simulink model "test1my"  (R2024b)
settings: Solver=VariableStepAuto  StartTime=0.0  StopTime=0.5  RelTol=1e-3
undefined symbols (not defined in the file): Ion, Lithium
libraries: spsSeriesRLCBranchLib x7, spsVoltageMeasurementLib x5, spsMosfetLib x3, spsCurrentMeasurementLib x2, spsPVArrayLib x2, spsBatteryLib x1, spsBreakerLib x1, spsDiodeLib x1, slpidlib x1, spsTriangleGeneratorLib x1, sps_lib x1
settings Model: Creator=pansi  LastModifiedBy=ASUS

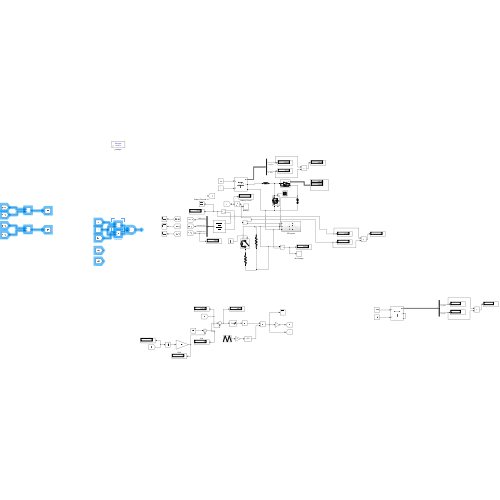
[thumbnail: Simulink's stored preview of the top-level diagram]
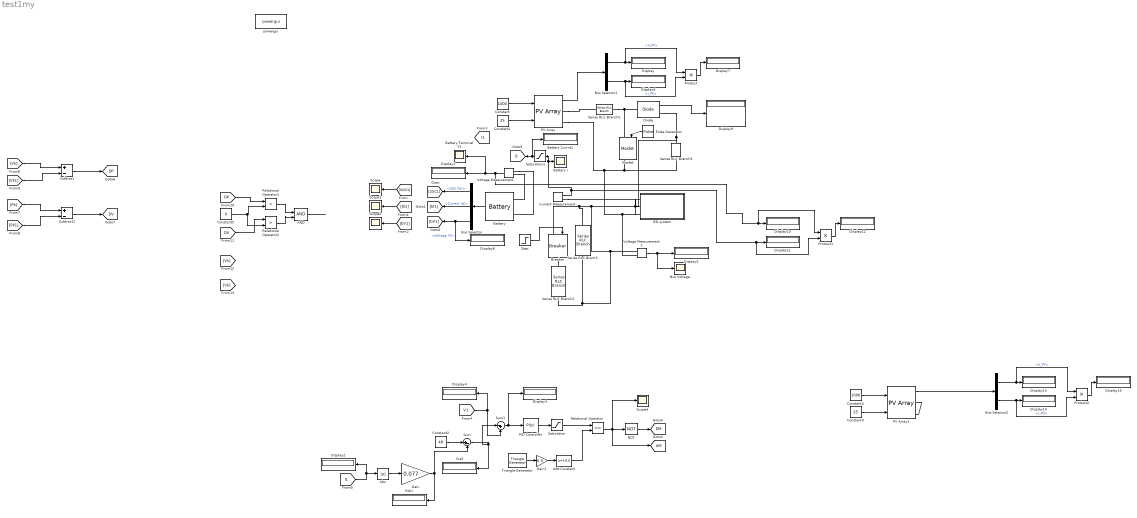
== system test1my ==
  AND : Logic  IconShape=distinctive  AllPortsSameDT=off  OutDataTypeStr=boolean
  Abs : Abs  SaturateOnIntegerOverflow=off
  Add Constant : Bias  Bias=+0.5  SaturateOnIntegerOverflow=off
  BD system : Subsystem
  Battery : spsBatteryLib/Battery  BatType=Lithium-Ion  NomV=48  NomQ=100  SOC=85  Batt_Tr=1  PresetModel=off  MaxQ=111  MinV=40  FullV=54.75  Dis_rate=20  R=0.05  Normal_OP=100  expZone=[51.6,10]
  Battery Currnt1 : Display
  Battery I : Scope
  Battery Terminal V1 : Scope
  Breaker : spsBreakerLib/Breaker  InitialState=0  SwitchingTimes="[1/60  5/60]"  External=on  BreakerResistance=0.01  SnubberResistance=1e6  SnubberCapacitance=inf  Measurements=None  MoreParameters=on  NoBreakLoop=off
  Bus Selector : BusSelector  OutputSignals=SOC (%),Current (A),Voltage (V)
  Bus Selector1 : BusSelector  OutputSignals=V_PV,I_PV
  Bus Selector2 : BusSelector  OutputSignals=V_PV,I_PV
  Bus Voltage : Scope
  Constant : Constant  Value=1000
  Constant1 : Constant  Value=25
  Constant2 : Constant  Value=48
  Constant3 : Constant  Value=1000
  Constant4 : Constant  Value=25
  Constant5 : Constant  Value=0
  Current Measurement : spsCurrentMeasurementLib/Current Measurement  PhasorSimulation=off  OutputType=Complex  PSBequivalent=0
  Diode : spsDiodeLib/Diode  Ron=0.001  Lon=0  Vf=0.8  IC=0  UseSnubber=0  Rs=500  Cs=250e-9  Measurements=on
  Display{,1..15} (16 alike) : Display
  Gain : Gain  Gain=0.077
  Gain1 : Gain  Gain=0.5
  Mosfet : spsMosfetLib/Mosfet  Ron=0.001  Lon=0  Rd=0.01  Vfd=0.8  IC=0  Rs=1e4  Cs=inf  Measurements=on
  NOT : Logic  Operator=NOT  IconShape=distinctive  AllPortsSameDT=off  OutDataTypeStr=boolean
  PID Controller : slpidlib/PID Controller  Controller=PI  Form=Parallel  TimeDomain=Discrete-time  UseExternalTs=off  SampleTime=-1  IntegratorMethod=Forward Euler  FilterMethod=Forward Euler  ControllerParametersSource=internal  P=0.5  I=100  UseKiTs=off  D=0  UseExternalDerivativeSource=off  N=100  UseFilter=on  TunerSelectOption=Transfer Function Based (PID Tuner App)  InitialConditionSource=internal  InitialConditionForIntegrator=0  InitialConditionForFilter=0  DifferentiatorICPrevScaledInput=0  ExternalReset=none  TrackingMode=off  Kt=1  LimitOutput=on  SatLimitsSource=internal  UpperSaturationLimit=1  LowerSaturationLimit=0  LinearizeAsGain=on  AntiWindupMode=none  Kb=1  LimitIntegrator=off  UpperIntegratorSaturationLimit=inf  LowerIntegratorSaturationLimit=-inf  POutMin=[]  POutMax=[]  IOutMin=[]  IOutMax=[]  DOutMin=[]  DOutMax=[]  NOutMin=[]  NOutMax=[]  SumOutMin=[]  SumOutMax=[]  SaturationOutMin=[]  SaturationOutMax=[]  PParamMin=[]  PParamMax=[]  IParamMin=[]  IParamMax=[]  DParamMin=[]  DParamMax=[]  NParamMin=[]  NParamMax=[]  KbParamMin=[]  KbParamMax=[]  KtParamMin=[]  KtParamMax=[]  KbOutMin=[]  KbOutMax=[]  KtOutMin=[]  KtOutMax=[]  IntegratorOutMin=[]  IntegratorOutMax=[]  FilterOutMin=[]  FilterOutMax=[]  SumI1OutMin=[]  SumI1OutMax=[]  SumI2OutMin=[]  SumI2OutMax=[]  SumI3OutMin=[]  SumI3OutMax=[]  SumI4OutMin=[]  SumI4OutMax=[]  SumDOutMin=[]  SumDOutMax=[]  DifferentiatorOutMin=[]  DifferentiatorOutMax=[]  FilterDiffOutCoefMin=[]  FilterDiffOutCoefMax=[]  ReciprocalOutMin=[]  ReciprocalOutMax=[]  SumDenOutMin=[]  SumDenOutMax=[]  SumNumOutMin=[]  SumNumOutMax=[]  DivideOutMin=[]  DivideOutMax=[]  UdiffTsProdOutMin=[]  UdiffTsProdOutMax=[]  NTsProdOutMin=[]  NTsProdOutMax=[]  UintegralTsProdOutMin=[]  UintegralTsProdOutMax=[]  UngainTsProdOutMin=[]  UngainTsProdOutMax=[]  ClampingZeroOutDataTypeStr=Inherit: Inherit via back propagation  ClampingZeroOutMin=[]  ClampingZeroOutMax=[]  FilterDenConstantOutDataTypeStr=Inherit: Inherit via back propagation  FilterDenConstantOutMin=[]  FilterDenConstantOutMax=[]  PCopyOutDataTypeStr=Inherit: Inherit via back propagation  PCopyOutMin=[]  PCopyOutMax=[]  NCopyOutDataTypeStr=Inherit: Inherit via back propagation  NCopyOutMin=[]  NCopyOutMax=[]  IntegratorContinuousStateAttributes=''  IntegratorStateMustResolveToSignalObject=off  IntegratorRTWStateStorageClass=Auto  FilterContinuousStateAttributes=''  FilterStateMustResolveToSignalObject=off  FilterRTWStateStorageClass=Auto  ParallelPVariant=InternalParameters  IdealPVariant=Disabled  IVariant=InternalParameters  DVariant=Disabled  IntegratorVariant=Discrete  SatVariant=Enabled  AWVariant=Passthrough  PCopyVariant=Disabled  TRVariant=Disabled  FdbkBlocksVariant=Forward  IdealPFdbkVariant=Disabled  SatFdbkVariant=Disabled  DerivativeFilterVariant=Disabled  NVariant=Disabled  NCopyVariant=Disabled_SignalSpec  FilterICVariant=Disabled  IntegratorICVariant=InternalICs  ExternalResetVariant=Disabled  TRSumVariant=Passthrough  SumFdbkVariant=Disabled  SumVariant=Sum_PI  TsampFilterVariant=InternalTs  TsampNgainVariant=Passthrough  TsampIntegralVariant=Disabled_SignalSpec  ExternalSaturationOutDataTypeStr=Inherit: Same as second input  DerivativeSourceVariant=Disabled  PreIntVariant=InternalPreInt
  PV Array : spsPVArrayLib/PV Array  Npar=5  Nser=1  PlotType=array @ 1000 W/m2 & specified temperatures  S_vec="[ 1000  500  100 ]"  Temp_C_vec="[ 45 25  ]"  ModuleName=User-defined  PlotWhenSelected=off  Pm=200.143  Ncell=60  Voc=32.9  Isc=8.21  Vm=26.3  Im=7.61  beta_Voc_pc=-0.123  alpha_Isc_pc=0.0032  beta_Voc=-0.040467  alpha_Isc=0.00026272  IL=8.2568  I0=9.0626e-16  nI=0.58154  Rsh=84.0292  Rs=0.47867  RobustModel=off  RobustCellTemperature=313.3991  BAL=off  Tc=1e-6  Tfilter=5e-5
  PV Array1 : spsPVArrayLib/PV Array  Npar=5  Nser=1  PlotType=array @ 1000 W/m2 & specified temperatures  S_vec="[ 1000  500  100 ]"  Temp_C_vec="[ 45 25  ]"  ModuleName=User-defined  PlotWhenSelected=off  Pm=200.143  Ncell=60  Voc=48  Isc=8.21  Vm=26.3  Im=7.61  beta_Voc_pc=-0.123  alpha_Isc_pc=0.0032  beta_Voc=-0.05904  alpha_Isc=0.00026272  IL=8.7965  I0=9.8099e-16  nI=0.8477  Rsh=16298.6629  Rs=2.539  RobustModel=off  RobustCellTemperature=313.3991  BAL=off  Tc=1e-6  Tfilter=5e-5
  Product : Product
  Product1 : Product
  Product2 : Product
  Pulse Generator : DiscretePulseGenerator  PulseType=Time based  Period=0.0001  PulseWidth=45.2
  RdxI : Display
  Relational Operator : RelationalOperator  Operator=<=  OutDataTypeStr=boolean  RndMeth=Simplest  InputSameDT=off
  Relational Operator1 : RelationalOperator  Operator=>  OutDataTypeStr=boolean  RndMeth=Simplest  InputSameDT=off
  Relational Operator2 : RelationalOperator  Operator=>  OutDataTypeStr=boolean  RndMeth=Simplest  InputSameDT=off
  Saturation : Saturate  UpperLimit=0.9  LowerLimit=0.1
  Saturation1 : Saturate  UpperLimit=31.5  LowerLimit=-31.5
  Scope{,1..2,4} (4 alike) : Scope
  Series RLC Branch : spsSeriesRLCBranchLib/Series RLC Branch  LConnTagsString=__new0  RConnTagsString=__new0  BranchType=R  Resistance=2.3  Inductance=1e-3  SetiL0=off  InitialCurrent=0  Capacitance=1e-6  Setx0=off  InitialVoltage=0  Measurements=None
  Series RLC Branch1 : spsSeriesRLCBranchLib/Series RLC Branch  LConnTagsString=__new0  RConnTagsString=__new0  BranchType=R  Resistance=2.3  Inductance=1e-3  SetiL0=off  InitialCurrent=0  Capacitance=1e-6  Setx0=off  InitialVoltage=0  Measurements=None
  Series RLC Branch2 : spsSeriesRLCBranchLib/Series RLC Branch  LConnTagsString=__new0  RConnTagsString=__new0  BranchType=L  Resistance=1  Inductance=100e-6  SetiL0=off  InitialCurrent=0  Capacitance=1e-6  Setx0=off  InitialVoltage=0  Measurements=None
  Series RLC Branch3 : spsSeriesRLCBranchLib/Series RLC Branch  LConnTagsString=__new0  RConnTagsString=__new0  BranchType=RC  Resistance=0.01  Inductance=1e-3  SetiL0=off  InitialCurrent=0  Capacitance=2000e-6  Setx0=off  InitialVoltage=0  Measurements=None
  Step : Step  Time=0.2  SampleTime=0
  Subtract : Sum  Inputs=+-
  Subtract1 : Sum  Inputs=+-
  Sum : Sum  Inputs=|+-
  Sum1 : Sum  Inputs=|-+
  Triangle Generator : spsTriangleGeneratorLib/Triangle Generator  Freq=20000  Phase=0  Ts=1e-5
  Voltage Measurement : spsVoltageMeasurementLib/Voltage Measurement  PhasorSimulation=off  OutputType=Complex  PSBequivalent=0
  Voltage Measurement1 : spsVoltageMeasurementLib/Voltage Measurement  PhasorSimulation=off  OutputType=Complex  PSBequivalent=0
  Vref : Display
  powergui : sps_lib/powergui  Priority=1  SimulationMode=Discrete  SampleTime=1e-6  frequency=60  Iterations=50  frequencyindice=0  Pbase=100e6  ErrMax=1e-4  UnitsV=kV  UnitsW=MW  buscounter=0  FunctionMessages=off  echomessages=off  EnableUseOfTLC=off  CurrentSourceSwitches=off  DisableSnubberDevices=off  DisableRonSwitches=off  DisableVfSwitches=off  DisplayEquations=off  AutomaticDiscreteSolvers=off  SolverType=Tustin/Backward Euler (TBE)  Interpol=off  ExternalGateDelay=off  methode=off  Ts=100  x0status=blocks  SPID=on  SwTol=0  HookPort=off  NonlinearTolerance=1e-4  nMaxIteration=100  ContinueOnMaxIteration=off  RestoreLinks=warning  ResistiveCurrentMeasurement=off  Frange=[0:2:500]  Ylog=off  Xlog=on  ShowGrid=off  save=off  variable=ZData  structure=0  ZoomFFT=off  StartTime=0.0  cycles=1  DisplayStyle=1  fundamental=60  FreqAxis=off  MaxFrequency=1000  frequencyindicesteady=1  RmsSteady=1  display=off
  tag scope: DM=global, DP=global, DV=global, I1=global, UM=global
  wires:
  Triangle Generator/1 -> Gain1/1
  [bV1] -> Scope2/1
  NOT/1 -> [DM]
  [SOC1] -> Scope/1
  Bus Selector/3 -> Display8/1, [bV1]  "<Voltage (V)>"
  Bus Selector/1 -> [SOC1]  "<SOC (%)>"
  [V1] -> Sum1/2, Display4/1
  Sum1/1 -> Display3/1, PID Controller/1
  Abs/1 -> Gain/1
  Voltage Measurement/1 -> Product1/1, Display10/1, Battery Terminal V1/1, Display1/1
  Battery/1 -> Bus Selector/1
  Constant/1 -> PV Array/1
  [bI1] -> Scope1/1
  Relational Operator/1 -> Scope4/1, [UM], NOT/1
  Gain1/1 -> Add Constant/1
  Constant2/1 -> Sum/1
  Bus Selector/2 -> [bI1]  "<Current (A)>"
  Sum/1 -> Sum1/1, Vref/1
  Gain/1 -> Sum/2, RdxI/1
  Add Constant/1 -> Relational Operator/2
  Voltage Measurement1/1 -> Bus Voltage/1, Display5/1
  PV Array/1 -> Bus Selector1/1
  Bus Selector1/1 -> Product/1, Display/1  "<V_PV>"
  Bus Selector1/2 -> Product/2, Display6/1  "<I_PV>"
  PID Controller/1 -> Saturation/1
  Saturation/1 -> Relational Operator/1
  Current Measurement/1 -> Saturation1/1, Battery I/1, Product1/2, Display11/1
  Product/1 -> Display7/1
  [I1] -> Display2/1, Abs/1
  Step/1 -> Breaker/1
  Constant1/1 -> PV Array/2
  Pulse Generator/1 -> Mosfet/1
  Product1/1 -> Display12/1
  Diode/1 -> Display9/1
  Saturation1/1 -> Battery Currnt1/1, [I1]
  Constant3/1 -> PV Array1/1
  Product2/1 -> Display15/1
  Constant4/1 -> PV Array1/2
  PV Array1/1 -> Bus Selector2/1
  Bus Selector2/1 -> Product2/1, Display13/1  "<V_PV>"
  Bus Selector2/2 -> Product2/2, Display14/1  "<I_PV>"
  [Vk1] -> Subtract/2
  Constant5/1 -> Relational Operator2/2, Relational Operator1/2
  [Pk1] -> Subtract1/2
  [Pk] -> Subtract1/1
  [Vk] -> Subtract/1
  AND/1 -> ?
  Subtract/1 -> [DP]
  [DV] -> Relational Operator2/1
  Relational Operator1/1 -> AND/1
  Subtract1/1 -> [DV]
  Relational Operator2/1 -> AND/2
  [DP] -> Relational Operator1/1
  connections:
  Diode/RConn1 -- BD system/LConn3 -- Series RLC Branch/RConn1 -- Series RLC Branch1/RConn1 -- Voltage Measurement1/LConn1 -- Breaker/LConn1 -- Series RLC Branch/LConn1 -- Series RLC Branch3/LConn1
  Voltage Measurement/LConn1 -- Battery/LConn1
  Breaker/RConn1 -- Series RLC Branch1/LConn1
  Series RLC Branch2/RConn1 -- Mosfet/LConn1 -- Diode/LConn1
  PV Array/RConn1 -- Series RLC Branch2/LConn1
  PV Array/RConn2 -- Voltage Measurement1/LConn2 -- BD system/LConn1 -- Mosfet/RConn1 -- Series RLC Branch3/RConn1
  Current Measurement/RConn1 -- BD system/LConn2
  Voltage Measurement/LConn2 -- Battery/LConn2
  PV Array1/RConn1 -- PV Array1/RConn2

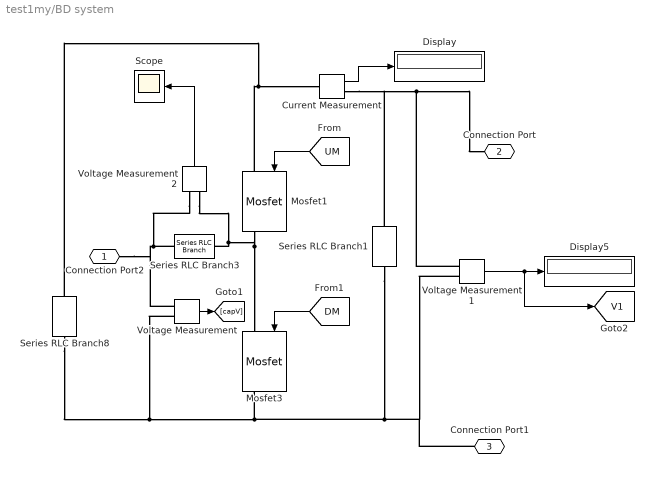
== system test1my/BD system ==
  Current Measurement : spsCurrentMeasurementLib/Current Measurement  PhasorSimulation=off  OutputType=Complex  PSBequivalent=0
  Display : Display
  Display5 : Display
  Mosfet1 : spsMosfetLib/Mosfet  Ron=0.1  Lon=0  Rd=0.01  Vfd=0  IC=0  Rs=1e6  Cs=inf  Measurements=on
  Mosfet3 : spsMosfetLib/Mosfet  Ron=0.1  Lon=0  Rd=0.01  Vfd=0  IC=0  Rs=1e6  Cs=inf  Measurements=on
  Scope : Scope
  Series RLC Branch1 : spsSeriesRLCBranchLib/Series RLC Branch  LConnTagsString=__new0  RConnTagsString=__new0  BranchType=C  Resistance=1  Inductance=1e-3  SetiL0=off  InitialCurrent=0  Capacitance=470e-6  Setx0=off  InitialVoltage=0  Measurements=None
  Series RLC Branch3 : spsSeriesRLCBranchLib/Series RLC Branch  LConnTagsString=__new0  RConnTagsString=__new0  BranchType=L  Resistance=1  Inductance=10e-6  SetiL0=off  InitialCurrent=0  Capacitance=1e-6  Setx0=off  InitialVoltage=0  Measurements=None
  Series RLC Branch8 : spsSeriesRLCBranchLib/Series RLC Branch  LConnTagsString=__new0  RConnTagsString=__new0  BranchType=RC  Resistance=1  Inductance=1e-3  SetiL0=off  InitialCurrent=0  Capacitance=1500e-6  Setx0=off  InitialVoltage=0  Measurements=None
  Voltage Measurement : spsVoltageMeasurementLib/Voltage Measurement  PhasorSimulation=off  OutputType=Complex  PSBequivalent=0
  Voltage Measurement1 : spsVoltageMeasurementLib/Voltage Measurement  PhasorSimulation=off  OutputType=Complex  PSBequivalent=0
  Voltage Measurement2 : spsVoltageMeasurementLib/Voltage Measurement  PhasorSimulation=off  OutputType=Complex  PSBequivalent=0
  Connection Port2 : PMIOPort  Side=Left
  Connection Port : PMIOPort  Port=2  Side=Left
  Connection Port1 : PMIOPort  Port=3  Side=Left
  tag scope: V1=global
  wires:
  Voltage Measurement1/1 -> [V1], Display5/1
  [UM] -> Mosfet1/1
  Voltage Measurement/1 -> [capV]
  Current Measurement/1 -> Display/1
  [DM] -> Mosfet3/1
  Voltage Measurement2/1 -> Scope/1
  connections:
  Voltage Measurement2/LConn2 -- Mosfet3/LConn1 -- Mosfet1/RConn1 -- Series RLC Branch3/RConn1
  Voltage Measurement1/LConn1 -- Current Measurement/RConn1 -- Series RLC Branch1/LConn1 -- Connection Port/RConn1
  Mosfet1/LConn1 -- Series RLC Branch8/LConn1 -- Current Measurement/LConn1
  Voltage Measurement/LConn2 -- Connection Port1/RConn1 -- Voltage Measurement1/LConn2 -- Series RLC Branch1/RConn1 -- Mosfet3/RConn1 -- Series RLC Branch8/RConn1
  Series RLC Branch3/LConn1 -- Connection Port2/RConn1 -- Voltage Measurement/LConn1 -- Voltage Measurement2/LConn1
